simulink model "ADU_Integration_Y2016_simulation"  (R2016b)
settings: Solver=FixedStepDiscrete  StartTime=240  StopTime=300  FixedStep=0.01  RelTol=1e-3  EnableMultiTasking=on
PostLoadFcn:
  | , if any(exist('dsrtsu_mdlpostloadfcn', 'file') == [2, 3, 6]), try dsrtsu_mdlpostloadfcn('Execute', bdroot); catch fprintf('Error in PostLoadFcn (dsrtsu_mdlpostloadfcn) for model "%s":\n %s\n', bdroot, lasterr); end, end,
InitFcn:
  | load 'data/chi2_dat';
  | load 'data/innerLine_struct';
  | load 'data/middleLine_struct';
  | load 'data/outerLine_struct';
  | load 'data/innerLine';
  | load 'data/middleLine';
  | load 'data/outerLine';
  | load 'data/landmarks_patac_schimmel_ccw';
  | load 'data/patac_navi_array';
  | load 'data/sensor';
  | load 'data/map_struct';
  | addpath map_src
  | Integration_Parameter;
  | load 'TestData_001';
values from neighbouring files (symbols this model uses):
  TestData_001 =     [TestData_001.mat]
undefined symbols (not defined in the file or in its folder): a, chi2_dat, innerLine, landmarks_patac_schimmel_ccw, middleLine, outerLine, patac_navi_array, StartNum
libraries: simulink x36, rtican x1
(part 10 of 20)

== stateflow chart ADU_Integration_Y2016_simulation/Fusion_Model/Fusion_Block/Global_Fusion/Fusion_Center ==
  state Fusion_Main [parallel]
    settings: executionOrder=2
    state D
    (default) -> D
    D -> (junction 4544)
    (junction 4544) -> (junction 4092) : {
        | FusDataIni();
        | FusTrackPredict();
        | MeasurementsGen();
        | FusTrackUpdate();
        | FusTrackIni();
        | }
    (junction 4092) -> (junction 4091) : {
        | Num_Trg=TrackCounter;
        | LastCalTime=Sensor_sampleTime;
        | }
    (junction 4091) -> (junction 4983) [order 1] : [RollCount<=2]
    (junction 4091) -> (junction 4987) [order 2] : {
        | RollCount=0;
        | }
    (junction 4983) -> (junction 4985) : {
        | RollCount++;
        | }
    (junction 4985) -> (junction 4987)
    (junction 4987) -> Fusion_Main
  state Set_Data_Source(data) [function]
    (default) -> (junction 1370)
    (junction 1370) -> (junction 1371) : {
        | DataSource = data;
        | }
  state DataSet [parallel]
    settings: executionOrder=1
    state C
    (default) -> C
    C -> (junction 5010)
    (junction 5010) -> (junction 5011) [order 1] : cal%Camera_Update
    (junction 5010) -> (junction 5015) [order 2]
    (junction 5011) -> (junction 5013) : {
        | Set_Data_Source(1);
        | Set_sampleTime(Camera_RxTime);
        | }
    (junction 5015) -> (junction 5017) [order 1] : cal1%SRR Update
    (junction 5015) -> (junction 5021) [order 2]
    (junction 5017) -> (junction 5019) : {
        | Set_Data_Source(3);
        | Set_sampleTime(SRR_RxTime);
        | }
    (junction 5021) -> (junction 5023) [order 1] : cal2%ESR Update
    (junction 5021) -> (junction 5027) [order 2]
    (junction 5023) -> (junction 5025) : {
        | Set_Data_Source(2);
        | Set_sampleTime(ESR_RxTime);
        | }
    (junction 5025) -> (junction 5027)
    (junction 5019) -> (junction 5025)
    (junction 5013) -> (junction 5019)
    (junction 5027) -> (junction 5047)
    (junction 5047) -> DataSet
  state Set_sampleTime(data) [function]
    (default) -> (junction 1375)
    (junction 1375) -> (junction 1376) : {
        | Sensor_sampleTime = data;
        | }
  state FusDataIni [function]
    (default) -> (junction 4085)
    (junction 4085) -> (junction 4086) : {
        | deltaT=Sensor_sampleTime-LastCalTime;ExistID=0;
        | k=0;n=0;m=0;FusDataOut=0;
        | FusDataInternal=0;%Initial step
        | MeasureData=0;MD_Exist=0;UpdateTrackFlag=0;
        | DelectTrackFlag=0;TrackCounter=0;Num_Out=0;ScoreFlag=0;
        | }
    (junction 4086) -> (junction 4087)
  state FusTrackPredict [function]
    state [RangeX,VelX,RangeY,VelY,P11,P12,P13,P14,P21,P22,P23,P24,P31,P32,P33,P34,P41,P42,P43,... [function]
      P44] = Forecast(Pre_x,Pre_vx,Pre_y,Pre_vy,deltaT,pre_p11,pre_p12,pre_p13,pre_p14,pre_p21,...
      pre_p22,pre_p23,pre_p24,pre_p31,pre_p32,pre_p33,pre_p34,pre_p41,pre_p42,pre_p43,pre_p44)
    (default) -> (junction 3932)
    (junction 3932) -> (junction 3933) [order 1] : [k<Num_Trg]
    (junction 3933) -> (junction 3934) [order 1] : [FusDataInternal_temp[k][0]!=0]
    (junction 3935) -> (junction 3932) : {
        | k++;
        | }
    (junction 3932) -> (junction 3937) [order 2] : {
        | Num_Trg=n;
        | n=0;
        | }
    (junction 3933) -> (junction 3935) [order 2]
    (junction 3934) -> (junction 3936) : {
        | [FusDataInternal[n][1],FusDataInternal[n][2],FusDataInternal[n][3],FusDataInternal[n][4],FusDataInternal[n][11],FusDataInternal[n][12],FusDataInternal[n][13],FusDataInternal[n][14],...
        | FusDataInternal[n][15],FusDataInternal[n][16],FusDataInternal[n][17],FusDataInternal[k][18],FusDataInternal[k][19],FusDataInternal[k][20],FusDataInternal[n][21],FusDataInternal[n][22],...
        | FusDataInternal[n][23],FusDataInternal[n][24],FusDataInternal[n][25],FusDataInternal[n][26]]=Forecast(FusDataInternal_temp[k][1],FusDataInternal_temp[k][2],FusDataInternal_temp[k][3],...
        | FusDataInternal_temp[k][4],deltaT,FusDataInternal_temp[k][11],FusDataInternal_temp[k][12],FusDataInternal_temp[k][13],FusDataInternal_temp[k][14],FusDataInternal_temp[k][15],FusDataInternal_temp[k][16],...
        | FusDataInternal_temp[k][17],FusDataInternal_temp[k][18],FusDataInternal_temp[k][19],FusDataInternal_temp[k][20],FusDataInternal_temp[k][21],FusDataInternal_temp[k][22],FusDataInternal_temp[k][23],...
        | FusDataInternal_temp[k][24],FusDataInternal_temp[k][25],FusDataInternal_temp[k][26]);%All fusion targets forecast,after this step, target number in FusDataInternal is the same as last calculation, but forecast with delta time
        | FusDataInternal[n][0]=FusDataInternal_temp[k][0];FusDataInternal[n][5]=FusDataInternal_temp[k][5];FusDataInternal[n][6]=FusDataInternal_temp[k][6];FusDataInternal[n][7]=FusDataInternal_temp[k][7];...
        | FusDataInternal[n][8]=FusDataInternal_temp[k][8];FusDataInternal[n][9]=FusDataInternal_temp[k][9];FusDataInternal[n][10]=FusDataInternal_temp[k][10];
        | FusDataInternal[n][27]=FusDataInternal_temp[k][27];FusDataInternal[n][28]=FusDataInternal_temp[k][28];FusDataInternal[n][29]=FusDataInternal_temp[k][29];
        | FusDataInternal[n][30]=FusDataInternal_temp[k][30];FusDataInternal[n][31]=FusDataInternal_temp[k][31];
        | n++;
        | }
    (junction 3936) -> (junction 3935)
  state MeasurementsGen [function]
    (default) -> (junction 4061) : {
        | k=0;
        | FusDataInternal_temp=0;
        | }
    (junction 4062) -> (junction 4063) [order 1] : [(k<64) ]
    (junction 4061) -> (junction 4062) [order 1] : [DataSource==2]%ESR Data Update
    (junction 4067) -> (junction 4062) : {
        | k++;
        | }
    (junction 4062) -> (junction 4069) [order 2]
    (junction 4063) -> (junction 4067) : {
        | MeasureData[k][0]=ESRData[k][0];
        | MeasureData[k][1]=ESRData[k][1];
        | MeasureData[k][2]=ESRData[k][2];
        | MeasureData[k][3]=0;MeasureData[k][4]=0;
        | MeasureData[k][5]=0;MeasureData[k][6]=0.1;
        | MeasureData[k][7]=0;MeasureData[k][8]=0;
        | MeasureData[k][9]=0.6;
        | }
    (junction 4061) -> (junction 4064) [order 2]
    (junction 4064) -> (junction 4547) [order 1] : [DataSource==3]%SRR Data Update
    (junction 4547) -> (junction 4549) [order 1] : [(k<40)]
    (junction 4551) -> (junction 4547) : {
        | k++;
        | }
    (junction 4064) -> (junction 4560) [order 2]
    (junction 4547) -> (junction 4068) [order 2]
    (junction 4549) -> (junction 4551) : {
        | MeasureData[k][0]=SRRData[k][0];
        | MeasureData[k][1]=SRRData[k][1];
        | MeasureData[k][2]=SRRData[k][2];
        | MeasureData[k][3]=SRRData[k][3];
        | MeasureData[k][4]=0;MeasureData[k][5]=0;
        | MeasureData[k][6]=1;MeasureData[k][7]=0;
        | MeasureData[k][8]=0;MeasureData[k][9]=1;
        | }
    (junction 4560) -> (junction 4065) [order 1] : [(k<25)]
    (junction 4066) -> (junction 4560) : {
        | k++;
        | }
    (junction 4065) -> (junction 4066) : {
        | MeasureData[k][0]=CameraData[k][0];MeasureData[k][1]=CameraData[k][1];
        | MeasureData[k][2]=CameraData[k][2];MeasureData[k][3]=CameraData[k][7];
        | MeasureData[k][4]=CameraData[k][4];MeasureData[k][5]=CameraData[k][3];
        | MeasureData[k][6]=0.3*CameraData[k][1];MeasureData[k][7]=0;
        | MeasureData[k][8]=0;MeasureData[k][9]=0.01;
        | }
    (junction 4560) -> (junction 4565) [order 2]
    (junction 4068) -> (junction 4565)
    (junction 4069) -> (junction 4068)
    (junction 4565) -> (junction 4070)
  state FusTrackUpdate [function]
    state [RangeX,VelX,RangeY,VelY,P11,P12,P13,P14,P21,P22,P23,P24,P31,P32,P33,P34,P41,P42,P43,... [function]
      P44] = Update(Pre_x,Pre_vx,Pre_y,Pre_vy,Mea_x,Mea_y,pre_p11,pre_p12,pre_p13,pre_p14,pre_p21,...
      pre_p22,pre_p23,pre_p24,pre_p31,pre_p32,pre_p33,pre_p34,pre_p41,pre_p42,pre_p43,pre_p44,R11,R12,R21,R22)
    state step1 [function]
      state Association_Update_step1 [function]
        (default) -> (junction 4252)
        (junction 4252) -> (junction 4253) [order 1] : [DataSource!=1]%Not Camera
        (junction 4253) -> (junction 4573) [order 1] : [DataSource!=2]%SRR
        (junction 4252) -> (junction 4254) [order 2] : {
            | ExistID=FusDataInternal[k][29];
            | }
        (junction 4253) -> (junction 4255) [order 2] : {
            | ExistID=FusDataInternal[k][27];
            | }
        (junction 4573) -> (junction 4575) : {
            | ExistID=FusDataInternal[k][28];
            | }
        (junction 4255) -> (junction 4254)
        (junction 4575) -> (junction 4255)
        (junction 4254) -> (junction 4257)
        (junction 4257) -> (junction 4256) [order 1] : [n<64]
        (junction 4256) -> (junction 4258) [order 1] : [(MeasureData[n][0]==ExistID) &&(MeasureData[n][10] == 0) &&(MeasureData[n][0] != 0)]
        (junction 4259) -> (junction 4257) : {
            | n++;
            | }
        (junction 4256) -> (junction 4259) [order 2]
        (junction 4257) -> (junction 4260) [order 2]
          settings: description=%not found last updata message
        (junction 4258) -> (junction 4261) : {
            | MD_Exist=MDCal(MeasureData[n][1],MeasureData[n][2],...
            | FusDataInternal[k][1],FusDataInternal[k][3],FusDataInternal[k][11],...
            | FusDataInternal[k][12],FusDataInternal[k][13],FusDataInternal[k][14],FusDataInternal[k][15],...
            | FusDataInternal[k][16],FusDataInternal[k][17],FusDataInternal[k][18],FusDataInternal[k][19],...
            | FusDataInternal[k][20],FusDataInternal[k][21],FusDataInternal[k][22],FusDataInternal[k][23],...
            | FusDataInternal[k][24],FusDataInternal[k][25],FusDataInternal[k][26],MeasureData[n][6],...
            | MeasureData[n][7],MeasureData[n][8],MeasureData[n][9]);
            | }
        (junction 4261) -> (junction 4260) [order 2] : %Not find exist measurement last time
          settings: description=%last measurement is out of range
        (junction 4261) -> (junction 4262) [order 1] : [MD_Exist<MD_Calib]
        (junction 4260) -> (junction 4263)
        (junction 4262) -> (junction 4727) : {
            | MeasureFoundNum=n;
            | [FusDataInternal_temp[k][1],FusDataInternal_temp[k][2],FusDataInternal_temp[k][3],FusDataInternal_temp[k][4],...
            | FusDataInternal_temp[k][11],FusDataInternal_temp[k][12],FusDataInternal_temp[k][13],FusDataInternal_temp[k][14],...
            | FusDataInternal_temp[k][15],FusDataInternal_temp[k][16],FusDataInternal_temp[k][17],FusDataInternal_temp[k][18],...
            | FusDataInternal_temp[k][19],FusDataInternal_temp[k][20],FusDataInternal_temp[k][21],FusDataInternal_temp[k][22],...
            | FusDataInternal_temp[k][23],FusDataInternal_temp[k][24],FusDataInternal_temp[k][25],FusDataInternal_temp[k][26]]=...
            | Update(FusDataInternal[k][1],FusDataInternal[k][2],FusDataInternal[k][3],FusDataInternal[k][4],...
            | MeasureData[MeasureFoundNum][1],MeasureData[MeasureFoundNum][2],...
            | FusDataInternal[k][11],FusDataInternal[k][12],FusDataInternal[k][13],FusDataInternal[k][14],...
            | FusDataInternal[k][15],FusDataInternal[k][16],FusDataInternal[k][17],FusDataInternal[k][18],...
            | FusDataInternal[k][19],FusDataInternal[k][20],FusDataInternal[k][21],FusDataInternal[k][22],...
            | FusDataInternal[k][23],FusDataInternal[k][24],FusDataInternal[k][25],FusDataInternal[k][26],...
            | MeasureData[MeasureFoundNum][6],MeasureData[MeasureFoundNum][7],MeasureData[MeasureFoundNum][8],MeasureData[MeasureFoundNum][9]);
            | FusDataInternal_temp[k][0]=FusDataInternal[k][0];FusDataInternal_temp[k][5]=FusDataInternal[k][5];FusDataInternal_temp[k][6]=FusDataInternal[k][6];
            | FusDataInternal_temp[k][8]=FusDataInternal[k][8];FusDataInternal_temp[k][9]=FusDataInternal[k][9];
            | FusDataInternal_temp[k][10]=FusDataInternal[k][10];FusDataInternal_temp[k][27]=FusDataInternal[k][27];
            | FusDataInternal_temp[k][28]=FusDataInternal[k][28];FusDataInternal_temp[k][29]=FusDataInternal[k][29];
            | FusDataInternal_temp[k][30]=FusDataInternal[k][30];FusDataInternal_temp[k][31]=FusDataInternal[k][31];
            | %Update track k with measurement (MeasureFoundNum)
            | UpdateTrackFlag[k]=1;%Track k is marked as updated
            | MeasureData[MeasureFoundNum][10]=1;%Measurement is marked as used
            | }
        (junction 4727) -> (junction 4728) [order 1] : [DataSource==1]%Camera
        (junction 4727) -> (junction 4264) [order 2] : {
            | FusDataInternal_temp[k][7]=FusDataInternal[k][7];
            | FusDataInternal_temp[k][6]=FusDataInternal[k][6];
            | }
        (junction 4728) -> (junction 4731) : {
            | FusDataInternal_temp[k][7]=MeasureData[MeasureFoundNum][10];
            | FusDataInternal_temp[k][6]=MeasureData[MeasureFoundNum][4];
            | }
        (junction 4264) -> (junction 4263)
        (junction 4731) -> (junction 4264)
        (junction 4263) -> (junction 4265)
      (default) -> (junction 4235) : {
          | k=0;ExistID=0;
          | %Gating and Association Step
          | }
      (junction 4235) -> (junction 4236) [order 1] : [k<Num_Trg]
      (junction 4240) -> (junction 4235) : {
          | n=0;k++;
          | MeasureFoundNum=0;
          | }
      (junction 4235) -> (junction 4239) [order 2]
      (junction 4236) -> (junction 4237) : {Association_Update_step1();}
      (junction 4237) -> (junction 4238) [order 1] : [UpdateTrackFlag[k]==1]
      (junction 4237) -> (junction 4240) [order 2]
      (junction 4238) -> (junction 4241) : {
          | UpdateSourceID();
          | }
      (junction 4241) -> (junction 4240)
    state step2 [function]
      state Association_Update_step2 [function]
        state gating [function]
          (default) -> (junction 4342)
          (junction 4342) -> (junction 4343) [order 1] : [m<64]
          (junction 4343) -> (junction 4344) [order 1] : [(MeasureData[m][0] !=0) &&...
              |  (MeasureData[m][10]==0)]
          (junction 4354) -> (junction 4342) : {
              | m++;
              | }
          (junction 4342) -> (junction 4351) [order 2]
          (junction 4343) -> (junction 4354) [order 2]
          (junction 4344) -> (junction 4348)
          (junction 4348) -> (junction 4346) [order 1] : [(MeasureData[m][1] <= FusDataInternal[k][1] + Rx3xgm) && ...
              |  (MeasureData[m][1] >= FusDataInternal[k][1] - Rx3xgm)  &&...
              |  (MeasureData[m][2] <= FusDataInternal[k][3] + Ry3xgm) && ...
              |  (MeasureData[m][2] >= FusDataInternal[k][3] - Ry3xgm)]
          (junction 4348) -> (junction 4355) [order 2]
          (junction 4346) -> (junction 4349) : {
              | MD_k_m=MDCal(MeasureData[m][1],MeasureData[m][2],...
              | FusDataInternal[k][1],FusDataInternal[k][3],FusDataInternal[k][11],...
              | FusDataInternal[k][12],FusDataInternal[k][13],FusDataInternal[k][14],FusDataInternal[k][15],...
              | FusDataInternal[k][16],FusDataInternal[k][17],FusDataInternal[k][18],FusDataInternal[k][19],...
              | FusDataInternal[k][20],FusDataInternal[k][21],FusDataInternal[k][22],FusDataInternal[k][23],...
              | FusDataInternal[k][24],FusDataInternal[k][25],FusDataInternal[k][26],MeasureData[m][6],...
              | MeasureData[m][7],MeasureData[m][8],MeasureData[m][9]);
              | }
          (junction 4349) -> (junction 4350) [order 1] : [MD_k_m<MD_min]
          (junction 4349) -> (junction 4352) [order 2]
          (junction 4350) -> (junction 4353) : {
              | MD_min=MD_k_m;
              | MeasureFoundFlag=1;
              | MeasureFoundNum=m;
              | }
          (junction 4353) -> (junction 4352)
          (junction 4352) -> (junction 4355)
          (junction 4355) -> (junction 4354)
        (default) -> (junction 4300)
        (junction 4300) -> (junction 4301) [order 1] : [(DataSource==2) || (DataSource==3)]%Radar(ESR and SRR)
        (junction 4300) -> (junction 4302) [order 2] : {
            | Ry3xgm=1;
            | }
        (junction 4301) -> (junction 4589) : {
            | Ry3xgm=1;
            | }
        (junction 4302) -> (junction 4303) [order 1] : [FusDataInternal[k][1] >= 0]
        (junction 4589) -> (junction 4590) [order 1] : [FusDataInternal[k][1]>=0]
        (junction 4302) -> (junction 4304) [order 2] : {
            | Rx3xgm=-0.3*FusDataInternal[k][1]+1;
            | }
        (junction 4589) -> (junction 4306) [order 2] : {
            | Rx3xgm=-0.15*FusDataInternal[k][1]+1;
            | }
        (junction 4303) -> (junction 4305) : {
            | Rx3xgm=0.3*FusDataInternal[k][1]+1;
            | }
        (junction 4590) -> (junction 4592) : {
            | Rx3xgm=0.15*FusDataInternal[k][1]+1;
            | }
        (junction 4305) -> (junction 4304)
        (junction 4306) -> (junction 4305)
        (junction 4592) -> (junction 4306)
        (junction 4304) -> (junction 4307)
        (junction 4307) -> (junction 4308) [order 1] : [UpdateTrackFlag[k]==0]
        (junction 4307) -> (junction 4315) [order 2]
        (junction 4308) -> (junction 4309) : {
            | gating();
            | }
        (junction 4309) -> (junction 4310) [order 1] : [MeasureFoundFlag ==1]
        (junction 4309) -> (junction 4311) [order 2] : {
            | UpdateTrackFlag[k]=0;
            | %Track k is not found updata measurement
            | }
        (junction 4310) -> (junction 4740) : {
            | [FusDataInternal_temp[k][1],FusDataInternal_temp[k][2],FusDataInternal_temp[k][3],FusDataInternal_temp[k][4],...
            | FusDataInternal_temp[k][11],FusDataInternal_temp[k][12],FusDataInternal_temp[k][13],FusDataInternal_temp[k][14],...
            | FusDataInternal_temp[k][15],FusDataInternal_temp[k][16],FusDataInternal_temp[k][17],FusDataInternal_temp[k][18],...
            | FusDataInternal_temp[k][19],FusDataInternal_temp[k][20],FusDataInternal_temp[k][21],FusDataInternal_temp[k][22],...
            | FusDataInternal_temp[k][23],FusDataInternal_temp[k][24],FusDataInternal_temp[k][25],FusDataInternal_temp[k][26]]=...
            | Update(FusDataInternal[k][1],FusDataInternal[k][2],FusDataInternal[k][3],FusDataInternal[k][4],...
            | MeasureData[MeasureFoundNum][1],MeasureData[MeasureFoundNum][2],...
            | FusDataInternal[k][11],FusDataInternal[k][12],FusDataInternal[k][13],FusDataInternal[k][14],...
            | FusDataInternal[k][15],FusDataInternal[k][16],FusDataInternal[k][17],FusDataInternal[k][18],...
            | FusDataInternal[k][19],FusDataInternal[k][20],FusDataInternal[k][21],FusDataInternal[k][22],...
            | FusDataInternal[k][23],FusDataInternal[k][24],FusDataInternal[k][25],FusDataInternal[k][26],...
            | MeasureData[MeasureFoundNum][6],MeasureData[MeasureFoundNum][7],MeasureData[MeasureFoundNum][8],MeasureData[MeasureFoundNum][9]);
            | FusDataInternal_temp[k][0]=FusDataInternal[k][0];FusDataInternal_temp[k][5]=FusDataInternal[k][5];FusDataInternal_temp[k][6]=FusDataInternal[k][6];
            | FusDataInternal_temp[k][8]=FusDataInternal[k][8];FusDataInternal_temp[k][9]=FusDataInternal[k][9];
            | FusDataInternal_temp[k][10]=FusDataInternal[k][10];FusDataInternal_temp[k][27]=FusDataInternal[k][27];
            | FusDataInternal_temp[k][28]=FusDataInternal[k][28];FusDataInternal_temp[k][29]=FusDataInternal[k][29];
            | FusDataInternal_temp[k][30]=FusDataInternal[k][30];FusDataInternal_temp[k][31]=FusDataInternal[k][31];%Update track k with measurement (MeasureFoundNum)
            | UpdateTrackFlag[k]=1;%Track k is marked as updated
            | MeasureData[MeasureFoundNum][10]=1;%Measurement is marked as used
            | }
        (junction 4311) -> (junction 4312) [order 1] : [c<32]
        (junction 4313) -> (junction 4311) : {c++;}
        (junction 4311) -> (junction 4316) [order 2] : {
            | c=0;
            | }
        (junction 4312) -> (junction 4313) : {
            | FusDataInternal_temp[k][c]=...
            | FusDataInternal[k][c];
            | }
        (junction 4740) -> (junction 4738) [order 1] : [DataSource==1]%Camera
        (junction 4738) -> (junction 4737) : {
            | FusDataInternal_temp[k][7]=MeasureData[MeasureFoundNum][10];
            | FusDataInternal_temp[k][6]=MeasureData[MeasureFoundNum][4];
            | }
        (junction 4740) -> (junction 4314) [order 2] : {
            | FusDataInternal_temp[k][7]=FusDataInternal[k][7];
            | FusDataInternal_temp[k][6]=FusDataInternal[k][6];
            | }
        (junction 4737) -> (junction 4314)
        (junction 4314) -> (junction 4316)
        (junction 4316) -> (junction 4315)
        (junction 4315) -> (junction 4317)
      (default) -> (junction 4285) : {
          | k=0;MD_min=8000;m=0;TrackCounter=0;
          | Rx3xgm=0;Ry3xgm=0;%Gating and Association Step
          | }
      (junction 4285) -> (junction 4286) [order 1] : [k<Num_Trg]
      (junction 4286) -> (junction 4287) [order 1] : [UpdateTrackFlag[k]==0]
      (junction 4288) -> (junction 4285) : {
          | k++;MeasureFoundFlag=0;m=0;
          | MD_min=8000;
          | }
      (junction 4285) -> (junction 4290) [order 2]
      (junction 4286) -> (junction 4288) [order 2]
      (junction 4287) -> (junction 4289) : {
          | Association_Update_step2();
          | UpdateSourceID();
          | }
      (junction 4289) -> (junction 4288)
    state MD = MDCal(MeasureRx,MeasureRy,PredictRx,PredictRy,P11,P12,... [function]
      P13,P14,P21,P22,P23,P24,P31,P32,P33,P34,P41,P42,P43,P44,R11,R12,R21,R22)
    state step3 [function]
      state FusTrackManagement [function]
        state ExistScoreCal [function]
          state OutSRRFOV= OutSRRFOV [function]
            (default) -> (junction 4680)
            (junction 4680) -> (junction 4710) [order 1] : [(FusDataInternal_temp[k][1]>=0)]
            (junction 4710) -> (junction 4712) [order 1] : [((FusDataInternal_temp[k][1])*(FusDataInternal_temp[k][1])+(FusDataInternal_temp[k][3])*(FusDataInternal_temp[k][3])>=60*60) && ...
                | ((FusDataInternal_temp[k][3]<FusDataInternal_temp[k][1]*tan(20*3.14/180)) && (FusDataInternal_temp[k][3]>-1*FusDataInternal_temp[k][1]*tan(20*3.14/180)))]
            (junction 4680) -> (junction 4709) [order 2]
            (junction 4710) -> (junction 4716) [order 2]
            (junction 4712) -> (junction 4714) : {
                | OutSRRFOV=1;
                | }
            (junction 4716) -> (junction 4709)
            (junction 4709) -> (junction 4719) : {
                | OutSRRFOV=0;
                | }
            (junction 4714) -> (junction 4719)
            (junction 4719) -> (junction 4722)
          state OutESRFOV= OutESRFOV [function]
            (default) -> (junction 4636)
            (junction 4636) -> (junction 4637) [order 1] : [(FusDataInternal_temp[k][1]<=0)]%Source is ESR and out of FOV
            (junction 4636) -> (junction 4638) [order 2]
            (junction 4637) -> (junction 4639)
            (junction 4638) -> (junction 4655) [order 1] : [(FusDataInternal_temp[k][1]>=60)]%LRR Mode
            (junction 4655) -> (junction 4639) [order 1] : [(FusDataInternal_temp[k][3]>FusDataInternal_temp[k][1]*tan(10*3.14/180)) || ...
                | (FusDataInternal_temp[k][3]<-1*FusDataInternal_temp[k][1]*tan(10*3.14/180))]
            (junction 4638) -> (junction 4657) [order 2]
            (junction 4655) -> (junction 4661) [order 2] : {
                | OutESRFOV = 0;
                | }
            (junction 4639) -> (junction 4641) : {
                | OutESRFOV = 1;
                | }
            (junction 4657) -> (junction 4669) [order 1] : [(FusDataInternal_temp[k][3]>FusDataInternal_temp[k][1]*tan(45*3.14/180)) || ...
                | (FusDataInternal_temp[k][3]<-1*FusDataInternal_temp[k][1]*tan(45*3.14/180))]%MRR Mode
            (junction 4657) -> (junction 4640) [order 2] : {
                | OutESRFOV = 0;
                | }
            (junction 4669) -> (junction 4670) : {
                | OutESRFOV = 1;
                | }
            (junction 4670) -> (junction 4640)
            (junction 4661) -> (junction 4670)
            (junction 4641) -> (junction 4661)
            (junction 4640) -> (junction 4642)
          state OutCameraFOV= OutCameraFOV [function]
            (default) -> (junction 4608)
            (junction 4608) -> (junction 4622) [order 1] : [(FusDataInternal_temp[k][1]<=0)]%Source is Camera and out of FOV
            (junction 4608) -> (junction 4628) [order 2]
            (junction 4622) -> (junction 4630)
            (junction 4628) -> (junction 4630) [order 1] : [(FusDataInternal_temp[k][3]>FusDataInternal_temp[k][1]*tan(20*3.14/180)) || ...
                | (FusDataInternal_temp[k][3]<-1*FusDataInternal_temp[k][1]*tan(20*3.14/180))]
            (junction 4628) -> (junction 4610) [order 2] : {
                | OutCameraFOV = 0;
                | }
            (junction 4630) -> (junction 4624) : {
                | OutCameraFOV = 1;
                | }
            (junction 4624) -> (junction 4610)
            (junction 4610) -> (junction 4612)
          state Blocked = CameraBlocked [function]
            (default) -> (junction 4437) : {
                | h = 0;
                | }
            (junction 4435) -> (junction 5000) [order 1] : [(MeasureData[h][0]!=0)&&...
                | (MeasureData[h][1]>0)]
            (junction 5000) -> (junction 4436) [order 1] : [(FusDataInternal_temp[k][1] >MeasureData[h][1]+2)&&...
                | (FusDataInternal_temp[k][1] <MeasureData[h][1]+20)&&...
                | (FusDataInternal_temp[k][3] <MeasureData[h][2] +1)&&...
                | (FusDataInternal_temp[k][3] >MeasureData[h][2] -1)]
            (junction 4437) -> (junction 4435) [order 1] : [h<25]
            (junction 4435) -> (junction 4438) [order 2]
            (junction 5000) -> (junction 5002) [order 2]
            (junction 4436) -> (junction 4440) : {
                | Blocked = 1;
                | }
            (junction 4438) -> (junction 4437) : {
                | h++;
                | }
            (junction 4437) -> (junction 4439) [order 2] : {
                | Blocked = 0;
                | }
            (junction 5002) -> (junction 4438)
            (junction 4440) -> (junction 4439)
            (junction 4439) -> (junction 4441)
          state ScoreIncrease [function]
            state CameraIncrease [function]
              (default) -> (junction 4883)
              (junction 4883) -> (junction 4886) : {
                  | FusDataInternal_temp[k][30]=...
                  | FusDataInternal_temp[k][30]+CameraScoreIn;
                  | FusDataInternal_temp[k][32]=7;
                  | }
              (junction 4886) -> (junction 4889)
            state SRRIncrease [function]
              (default) -> (junction 4901)
              (junction 4901) -> (junction 4902) : {
                  | FusDataInternal_temp[k][30]=...
                  | FusDataInternal_temp[k][30]+SRRScoreIn;
                  | FusDataInternal_temp[k][32]=8;
                  | }
              (junction 4902) -> (junction 4903)
            state ESRIncrease [function]
              (default) -> (junction 4908)
              (junction 4908) -> (junction 4914) [order 1] : [(FusDataInternal_temp[k][3]<10) &&...
                  |  (FusDataInternal_temp[k][3]>-10)]
              (junction 4914) -> (junction 4920) [order 1] : [(FusDataInternal_temp[k][3]<5) &&...
                  |  (FusDataInternal_temp[k][3]>-5)]
              (junction 4908) -> (junction 4909) [order 2] : {
                  | FusDataInternal_temp[k][30]=...
                  | FusDataInternal_temp[k][30]+ESRScoreIn;
                  | FusDataInternal_temp[k][32]=91;
                  | %Lateral Range is Far
                  | }
              (junction 4914) -> (junction 4924) [order 2] : {
                  | FusDataInternal_temp[k][30]=...
                  | FusDataInternal_temp[k][30]+ESRScoreIn;
                  | FusDataInternal_temp[k][32]=92;
                  | %Lateral Range is Middle
                  | }
              (junction 4920) -> (junction 4922) : {
                  | FusDataInternal_temp[k][30]=...
                  | FusDataInternal_temp[k][30]+ESRScoreIn;
                  | FusDataInternal_temp[k][32]=93;
                  | %Lateral Range is Near
                  | }
              (junction 4924) -> (junction 4909)
              (junction 4922) -> (junction 4924)
              (junction 4909) -> (junction 4910)
            (default) -> (junction 4755)
            (junction 4755) -> (junction 4762) [order 1] : [DataSource!=1]
            (junction 4762) -> (junction 4768) [order 1] : [DataSource!=2]
            (junction 4755) -> (junction 4764) [order 2] : {
                | CameraIncrease();
                | %Camera
                | }
            (junction 4762) -> (junction 4766) [order 2] : {
                | ESRIncrease();
                | %ESR
                | }
            (junction 4768) -> (junction 4771) : {
                | SRRIncrease();
                | %SRR
                | }
            (junction 4766) -> (junction 4764)
            (junction 4771) -> (junction 4766)
            (junction 4764) -> (junction 4775)
          state ScoreDecrease [function]
            (default) -> (junction 4778)
            (junction 4779) -> (junction 4780) [order 1] : [DataSource!=2]
            (junction 4778) -> (junction 4779) [order 1] : [DataSource!=1]
            (junction 4779) -> (junction 4782) [order 2] : {
                | FusDataInternal_temp[k][30]=...
                | FusDataInternal_temp[k][30]-ESRScoreDe;
                | FusDataInternal_temp[k][32]=13;
                | %ESR
                | }
            (junction 4780) -> (junction 4783) : {
                | FusDataInternal_temp[k][30]=...
                | FusDataInternal_temp[k][30]-SRRScoreDe;
                | FusDataInternal_temp[k][32]=14;
                | %SRR
                | }
            (junction 4778) -> (junction 4973) [order 2]
            (junction 4973) -> (junction 4975) [order 1] : [((FusDataInternal_temp[k][3]<3) && (FusDataInternal_temp[k][3]>-3))&&...
                | FusDataInternal_temp[k][1]<30]
            (junction 4973) -> (junction 4781) [order 2] : {
                | FusDataInternal_temp[k][30]=...
                | FusDataInternal_temp[k][30]-CameraFarScoreDe;
                | FusDataInternal_temp[k][32]=11;
                | %Camera
                | }
            (junction 4975) -> (junction 4977) : {
                | FusDataInternal_temp[k][30]=...
                | FusDataInternal_temp[k][30]-CameraNearScoreDe;
                | FusDataInternal_temp[k][32]=12;
                | %Camera
                | }
            (junction 4783) -> (junction 4782)
            (junction 4782) -> (junction 4977)
            (junction 4977) -> (junction 4781)
            (junction 4781) -> (junction 4784)
          (default) -> (junction 4401)
          (junction 4401) -> (junction 4400) [order 1] : [UpdateTrackFlag[k]==1]
          (junction 4400) -> (junction 4404) : {
              | ScoreIncrease();
              | ScoreFlag=6;
              | }
          (junction 4401) -> (junction 4402) [order 2]
          (junction 4402) -> (junction 4403) [order 1] : [(DataSource==1) && (OutCameraFOV()==1)]%Source is Camera and out of FOV
          (junction 4402) -> (junction 4406) [order 2]
          (junction 4403) -> (junction 4410) : {
              | FusDataInternal_temp[k][32]=5;
              | }
          (junction 4406) -> (junction 4407) [order 1] : [(DataSource==1) && (FusDataInternal_temp[k][1]>0) &&(CameraBlocked() ==1)]% Source is Camera, but is blocked by other object
          (junction 4406) -> (junction 4599) [order 2]
          (junction 4407) -> (junction 4409) : {
              | FusDataInternal_temp[k][32]=4;
              | }
          (junction 4599) -> (junction 4601) [order 1] : [(DataSource==2) && (OutESRFOV()==1)]%Source is ESR and out of FOV
          (junction 4599) -> (junction 4673) [order 2]
          (junction 4601) -> (junction 4652) : {
              | FusDataInternal_temp[k][32]=3;
              | }
          (junction 4673) -> (junction 4675) [order 1] : [(DataSource==3) && (OutSRRFOV()==1)] % Source is SRR and out of FOV
          (junction 4673) -> (junction 4408) [order 2] : {
              | ScoreDecrease();
              | }
          (junction 4675) -> (junction 4724) : {
              | FusDataInternal_temp[k][32]=2;
              | }
          (junction 4404) -> (junction 4405) [order 1] : [FusDataInternal_temp[k][30]>18]
          (junction 4404) -> (junction 4411) [order 2]
          (junction 4405) -> (junction 4412) : {
              | FusDataInternal_temp[k][30]=18;
              | }
          (junction 4724) -> (junction 4408)
          (junction 4652) -> (junction 4724)
          (junction 4412) -> (junction 4411)
          (junction 4409) -> (junction 4652)
          (junction 4411) -> (junction 4410)
          (junction 4410) -> (junction 4409)
          (junction 4408) -> (junction 4413)
        state OutputTrack [function]
          (default) -> (junction 4452)
          (junction 4452) -> (junction 4453) [order 1] : [FusDataInternal_temp[k][31]==0]%Not a confirmed track
          (junction 4453) -> (junction 4454) [order 1] : [FusDataInternal_temp[k][30]<15]
          (junction 4452) -> (junction 4455) [order 2]
          (junction 4453) -> (junction 4456) [order 2] : {
              | FusDataInternal_temp[k][31]=1;
              | %New confirmed track
              | }
          (junction 4454) -> (junction 4464) : {
              | TrackCounter++;
              | }
          (junction 4456) -> (junction 4455)
          (junction 4455) -> (junction 4457) : {
              | FusDataOut[Num_Out][0]=FusDataInternal_temp[k][0];FusDataOut[Num_Out][1]=FusDataInternal_temp[k][1];
              | FusDataOut[Num_Out][2]=FusDataInternal_temp[k][2];FusDataOut[Num_Out][3]=FusDataInternal_temp[k][3];
              | FusDataOut[Num_Out][4]=FusDataInternal_temp[k][4];FusDataOut[Num_Out][5]=0;FusDataOut[Num_Out][6]=FusDataInternal_temp[k][6];FusDataOut[Num_Out][8]=0;
              | FusDataOut[Num_Out][7]=FusDataInternal_temp[k][7];%Type
              | FusDataOut[Num_Out][10]=FusDataInternal_temp[k][11];FusDataOut[Num_Out][11]=FusDataInternal_temp[k][12];
              | FusDataOut[Num_Out][12]=FusDataInternal_temp[k][13];FusDataOut[Num_Out][13]=FusDataInternal_temp[k][14];FusDataOut[Num_Out][14]=FusDataInternal_temp[k][15];
              | FusDataOut[Num_Out][15]=FusDataInternal_temp[k][16];FusDataOut[Num_Out][16]=FusDataInternal_temp[k][17];FusDataOut[Num_Out][17]=FusDataInternal_temp[k][18];
              | FusDataOut[Num_Out][18]=FusDataInternal_temp[k][19];FusDataOut[Num_Out][19]=FusDataInternal_temp[k][20];FusDataOut[Num_Out][20]=FusDataInternal_temp[k][21];
              | FusDataOut[Num_Out][21]=FusDataInternal_temp[k][22];FusDataOut[Num_Out][22]=FusDataInternal_temp[k][23];FusDataOut[Num_Out][23]=FusDataInternal_temp[k][24];
              | FusDataOut[Num_Out][24]=FusDataInternal_temp[k][25];FusDataOut[Num_Out][25]=FusDataInternal_temp[k][26];
              | %Select outputs signals from Internal to output
              | TrackCounter++;Num_Out++;
              | }
          (junction 4457) -> (junction 4458) [order 1] : [FusDataInternal_temp[k][30]<=15]
          (junction 4458) -> (junction 4459) [order 1] : [FusDataInternal_temp[k][30]<=9]
          (junction 4457) -> (junction 4460) [order 2] : {
              | FusDataOut[Num_Out-1][9]=3;
              | %High confidence
              | }
          (junction 4458) -> (junction 4461) [order 2] : {
              | FusDataOut[Num_Out-1][9]=2;
              | %Speculative
              | }
          (junction 4459) -> (junction 4462) : {
              | FusDataOut[Num_Out-1][9]=1;
              | %High Speculative
              | }
          (junction 4461) -> (junction 4460)
          (junction 4462) -> (junction 4461)
          (junction 4460) -> (junction 4463)
          (junction 4464) -> (junction 4463)
          (junction 4463) -> (junction 4465)
        state Del_InternalTrack [function]
          (default) -> (junction 4485) : {
              | DelectTrackFlag[k]=1;%mean that track need to delect
              | IDUsedFlag[FusDataInternal_temp[k][0]]=0;%Reflash ID Used Flag
              | }
          (junction 4485) -> (junction 4486) [order 1] : [c<32]
          (junction 4487) -> (junction 4485) : {c++;}
          (junction 4485) -> (junction 4488) [order 2] : {
              | c=0;
              | TrackCounter++;
              | }
          (junction 4486) -> (junction 4487) : {
              | FusDataInternal_temp[k][c]=0;
              | }
        (default) -> (junction 4386)
        (junction 4386) -> (junction 4387) : {
            | ExistScoreCal();
            | }
        (junction 4387) -> (junction 4388) [order 1] : [FusDataInternal_temp[k][30]>=0]%Marks >=0
        (junction 4387) -> (junction 4389) [order 2] : {
            | Del_InternalTrack();
            | }
        (junction 4388) -> (junction 4390) : {
            | OutputTrack();
            | }
        (junction 4390) -> (junction 4389)
        (junction 4389) -> (junction 4391)
      (default) -> (junction 4376) : {
          | k=0;TrackCounter=0;
          | }
      (junction 4376) -> (junction 4377) [order 1] : [k<Num_Trg]
      (junction 4379) -> (junction 4376) : {
          | k++;
          | }
      (junction 4376) -> (junction 4378) [order 2]
      (junction 4377) -> (junction 4379) : {
          | FusTrackManagement();
          | }
    state UpdateSourceID [function]
      (default) -> (junction 4521)
      (junction 4521) -> (junction 4522) [order 1] : [UpdateTrackFlag[k]==0]
      (junction 4522) -> (junction 4523) [order 1] : [DataSource !=1]
      (junction 4523) -> (junction 4578) [order 1] : [DataSource !=2]
      (junction 4521) -> (junction 4525) [order 2]
      (junction 4522) -> (junction 4529) [order 2] : {
          | FusDataInternal_temp[k][29] = -1;
          | }
      (junction 4523) -> (junction 4526) [order 2] : {
          | FusDataInternal_temp[k][27] = -1;
          | }
      (junction 4578) -> (junction 4580) : {
          | FusDataInternal_temp[k][28] = -1;
          | }
      (junction 4525) -> (junction 4524) [order 1] : [DataSource!=1]%ESR or SRR
      (junction 4524) -> (junction 4583) [order 1] : [DataSource!=2]%SRR
      (junction 4525) -> (junction 4527) [order 2] : {
          | FusDataInternal_temp[k][29]=MeasureData[MeasureFoundNum][0];
          | FusDataInternal_temp[k][9]=1;
          | }
      (junction 4524) -> (junction 4528) [order 2] : {
          | FusDataInternal_temp[k][27]=MeasureData[MeasureFoundNum][0];
          | FusDataInternal_temp[k][9]=2;
          | }
      (junction 4583) -> (junction 4585) : {
          | FusDataInternal_temp[k][28]=MeasureData[MeasureFoundNum][0];
          | FusDataInternal_temp[k][9]=3;
          | }
      (junction 4580) -> (junction 4526)
      (junction 4528) -> (junction 4527)
      (junction 4526) -> (junction 4529)
      (junction 4585) -> (junction 4528)
      (junction 4529) -> (junction 4585)
      (junction 4527) -> (junction 4530)
    (default) -> (junction 4095)
    (junction 4095) -> (junction 4096) : {
        | step1();
        | step2();
        | step3();
        | }
    (junction 4096) -> (junction 4097)
  state FusTrackIni [function]
    state InPathFlag =ESRInPathJudge(x,y,R) [function]
    (default) -> (junction 3890) : {
        | k=0;
        | n=0;
        | m=0;
        | }
    (junction 3890) -> (junction 3891) [order 1] : [k<64]
    (junction 3891) -> (junction 4929) [order 1] : [(MeasureData[k][0] !=0) && (MeasureData[k][10]==0)]
        | %Measurement k not association with fuse track
    (junction 4929) -> (junction 4958) [order 1] : [(DataSource==1) || (DataSource==3)]
    (junction 4958) -> (junction 3892)
    (junction 3892) -> (junction 3893) : {LastFusID++;}
    (junction 3893) -> (junction 3894) [order 1] : [LastFusID<127]
    (junction 3903) -> (junction 3890) : {
        | k++;
        | LoopError=0;
        | }
    (junction 3890) -> (junction 3902) [order 2]
    (junction 3891) -> (junction 3903) [order 2]
    (junction 4929) -> (junction 4933) [order 2] : {
        | InPathFlag=ESRInPathJudge(MeasureData[k][1],...
        | MeasureData[k][2],Path_Radius)
        | }%ESR Data
    (junction 4935) -> (junction 4958)
    (junction 3897) -> (junction 3892) : {
        | LoopError++;
        | }
    (junction 3893) -> (junction 3895) [order 2] : {LastFusID=1;}
    (junction 3894) -> (junction 3896)
    (junction 3895) -> (junction 3896)
    (junction 3896) -> (junction 3898)
    (junction 4933) -> (junction 4935) [order 1] : [(InPathFlag==1) && (DataSource==2)]
    (junction 3898) -> (junction 3897) [order 2] : [LoopError<126 && (IDUsedFlag[LastFusID]==1)]
    (junction 3898) -> (junction 3899) [order 1] : [IDUsedFlag[LastFusID]==0]
    (junction 4933) -> (junction 4961) [order 2]
    (junction 3898) -> (junction 3904) [order 3]
    (junction 3899) -> (junction 3900) : {
        | FusDataInternal_temp[TrackCounter][0]=LastFusID;IDUsedFlag[LastFusID]=1;
        | FusDataInternal_temp[TrackCounter][1]=MeasureData[k][1];FusDataInternal_temp[TrackCounter][2]=0;FusDataInternal_temp[TrackCounter][3]=MeasureData[k][2];
        | FusDataInternal_temp[TrackCounter][4]=0;
        | FusDataInternal_temp[TrackCounter][5]=0;FusDataInternal_temp[TrackCounter][6]=0;FusDataInternal_temp[TrackCounter][7]=0;
        | FusDataInternal_temp[TrackCounter][8]=0;FusDataInternal_temp[TrackCounter][9]=DataSource;
        | FusDataInternal_temp[TrackCounter][10]=1;
        | FusDataInternal_temp[TrackCounter][11]=1;FusDataInternal_temp[TrackCounter][16]=1;FusDataInternal_temp[TrackCounter][21]=1;FusDataInternal_temp[TrackCounter][26]=1;
        | FusDataInternal_temp[TrackCounter][30]=5;FusDataInternal_temp[TrackCounter][31]=0;
        | }
    (junction 3900) -> (junction 3901) [order 1] : [DataSource!=1]
    (junction 3901) -> (junction 4741) [order 1] : [DataSource!=2]
    (junction 3900) -> (junction 3905) [order 2] : {
        | FusDataInternal_temp[TrackCounter][29]=MeasureData[k][0];
        | FusDataInternal_temp[TrackCounter][6]=MeasureData[k][4];
        | FusDataInternal_temp[TrackCounter][7]=MeasureData[k][5];
        | TrackCounter++;
        | }
    (junction 3901) -> (junction 3906) [order 2] : {
        | FusDataInternal_temp[TrackCounter][27]=MeasureData[k][0];
        | TrackCounter++;
        | }
    (junction 4741) -> (junction 4743) : {
        | FusDataInternal_temp[TrackCounter][28]=MeasureData[k][0];
        | TrackCounter++;
        | }
    (junction 4961) -> (junction 3903)
    (junction 3904) -> (junction 4961)
    (junction 3905) -> (junction 3904)
    (junction 3906) -> (junction 3905)
    (junction 4743) -> (junction 3906)
  data: data function_input double; data function_input double; Pre_x function_input; Pre_vx function_input; Pre_y function_input; Pre_vy function_input; deltaT function_input; pre_p11 function_input; pre_p12 function_input; pre_p13 function_input; pre_p14 function_input; pre_p21 function_input; pre_p22 function_input; pre_p23 function_input; pre_p24 function_input; pre_p31 function_input; pre_p32 function_input; pre_p33 function_input; pre_p34 function_input; pre_p41 function_input; pre_p42 function_input; pre_p43 function_input; pre_p44 function_input; RangeX function_output; VelX function_output; RangeY function_output; VelY function_output; P11 function_output; P12 function_output; P13 function_output; P14 function_output; P21 function_output; P22 function_output; P23 function_output; P24 function_output; P31 function_output; P32 function_output; P33 function_output; P34 function_output; P41 function_output; P42 function_output; P43 function_output; P44 function_output; Pre_x function_input; Pre_vx function_input; Pre_y function_input; Pre_vy function_input; Mea_x function_input; Mea_y function_input; pre_p11 function_input; pre_p12 function_input; pre_p13 function_input; pre_p14 function_input; pre_p21 function_input; pre_p22 function_input; pre_p23 function_input; pre_p24 function_input; pre_p31 function_input; pre_p32 function_input; pre_p33 function_input; pre_p34 function_input; pre_p41 function_input; pre_p42 function_input; pre_p43 function_input; pre_p44 function_input; R11 function_input; R12 function_input; R21 function_input; R22 function_input; RangeX function_output; VelX function_output; RangeY function_output; VelY function_output; P11 function_output; P12 function_output; P13 function_output; P14 function_output; P21 function_output; P22 function_output; P23 function_output; P24 function_output; P31 function_output; P32 function_output; P33 function_output; P34 function_output; P41 function_output; P42 function_output; P43 function_output; P44 function_output; MeasureRx function_input; MeasureRy function_input; PredictRx function_input; PredictRy function_input; P11 function_input; P12 function_input; P13 function_input; P14 function_input; P21 function_input; P22 function_input; P23 function_input; P24 function_input; P31 function_input; P32 function_input; P33 function_input; P34 function_input; P41 function_input; P42 function_input; P43 function_input; P44 function_input; MD function_output; R11 function_input; R12 function_input; R21 function_input; R22 function_input; h temporary double =0; OutSRRFOV function_output double; h temporary double =0; OutESRFOV function_output double; h temporary double =0; OutCameraFOV function_output double; h temporary double =0; Blocked function_output double; x function_input; InPathFlag function_output; y function_input; R function_input double size=1; ESRData input size=[64 4]; FusDataOut output double size=[127 26] =0; MeasureData local double size=[64 11] =0; Num_Trg output double size=1 =0; FusDataInternal_temp local double size=[127 33]; PowerMode local double size=1 =1; DisableCriteria local double size=1 =0; CameraStatus constant double size=1 =1; RadarStatus constant double size=1 =1; DataSource local double size=1; Sensor_sampleTime local double size=1; CameraData input size=[25 8]; n local double size=1 =0; k local double size=1 =0; FusDataInternal local double size=[127 33]; LastCalTime local double size=1 =240; MD_Exist local double size=1 =0; MD_Calib constant double =800; Rx3xgm local double; Ry3xgm local double; MD_min local double size=1 =2000; MeasureFoundFlag local double size=1 =0; MeasureFoundNum local double size=1 =0; UpdateTrackFlag local double size=127 =0; TrackCounter local double size=1 =0; m local double size=1 =0; DelectTrackFlag local double size=127 =0; Num_Out local double size=1 =0; c local double size=1 =0; LastFusID local double size=1 =0; ExistID local double size=1 =0; IDUsedFlag local double size=127 =0; MD_k_m local double size=1 =0; deltaT local double size=1 =0; LoopError local double size=1 =0; SRRData input size=[40 4]; Path_Radius input double; InPathFlag local double; ScoreFlag local double; RollCount output double; CameraFarScoreDe constant double =2; CameraNearScoreDe constant double =5; ESRScoreDe constant double =4; SRRScoreDe constant double =2; SRRScoreIn constant double =4; ESRScoreIn constant double =5; CameraScoreIn constant double =6; ESR_RxTime input double; SRR_RxTime input double; Camera_RxTime input double
  events: cal input EITHER_EDGE_EVENT; cal1 input EITHER_EDGE_EVENT; cal2 input EITHER_EDGE_EVENT

== stateflow chart ADU_Integration_Y2016_simulation/Fusion_Model/Fusion_Block/Side_Fusion/LF_SRR_CoordinateAlig ==
  state [rangeX,rangeY] = TemporalAligLF(range,azimuth,W,L,InstallAngLFSRR) [function]
  (default) -> (junction 95) : {
      | k=0;
      | LFSRR_Output=0;
      | }
  (junction 95) -> (junction 98) [order 1] : [k<10]
  (junction 98) -> (junction 104) [order 1] : [LFSRR_Input[k][0]!=0]
  (junction 101) -> (junction 95) : {
      | k++;
      | }
  (junction 95) -> (junction 96) [order 2] : {
      | SideFusion;
      | }
  (junction 98) -> (junction 101) [order 2]
  (junction 104) -> (junction 106) : {
      | LFSRR_Output[k][0]=LFSRR_Input[k][0];%Target ID
      | [LFSRR_Output[k][1],LFSRR_Output[k][2]]=TemporalAligLF(LFSRR_Input[k][1],LFSRR_Input[k][2],W,L,InstallAng*3.1415/180);
      | LFSRR_Output[k][3]=LFSRR_Input[k][4]; %Target DynamicMode
      | }
  (junction 106) -> (junction 101)
  data: range function_input; rangeX function_output; rangeY function_output; azimuth function_input; W function_input double size=1; L function_input double size=1; InstallAngLFSRR function_input double size=1; LFSRR_Input input double size=[10 5]; LFSRR_Output output double size=[10 4]; k local double size=1 =0; W constant double =1.8; L constant double =5.2; InstallAng constant double =63
  events: SRR_Trig input EITHER_EDGE_EVENT; SideFusion output FUNCTION_CALL_EVENT

== stateflow chart ADU_Integration_Y2016_simulation/Fusion_Model/Fusion_Block/Side_Fusion/LR_SRR_CoordinateAlig ==
  state [rangeX,rangeY] = TemporalAligLR(range,azimuth,W,L,InstallAngLRSRR) [function]
  (default) -> (junction 95) : {
      | k=0;
      | LRSRR_Output=0;
      | }
  (junction 95) -> (junction 98) [order 1] : [k<10]
  (junction 98) -> (junction 104) [order 1] : [LRSRR_Input[k][0]!=0]
  (junction 101) -> (junction 95) : {
      | k++;
      | }
  (junction 95) -> (junction 96) [order 2] : {
      | SideFusion;
      | }
  (junction 98) -> (junction 101) [order 2]
  (junction 104) -> (junction 106) : {
      | LRSRR_Output[k][0]=LRSRR_Input[k][0];%Target ID
      | [LRSRR_Output[k][1],LRSRR_Output[k][2]]=TemporalAligLR(LRSRR_Input[k][1],LRSRR_Input[k][2],W,L,InstallAng*3.1415/180);
      | LRSRR_Output[k][3]=LRSRR_Input[k][4]; %Target DynamicMode
      | }
  (junction 106) -> (junction 101)
  data: range function_input; rangeX function_output; rangeY function_output; azimuth function_input; W function_input double size=1; L function_input double size=1; InstallAngLRSRR function_input double size=1; LRSRR_Input input double size=[10 5]; LRSRR_Output output double size=[10 4]; k local double size=1 =0; L constant double =5.2; W constant double =1.8; InstallAng constant double =60
  events: SRR_Trig input EITHER_EDGE_EVENT; SideFusion output FUNCTION_CALL_EVENT

== stateflow chart ADU_Integration_Y2016_simulation/LogData/Vision_Target/Chart1 ==
  (default) -> (junction 13)
  (junction 13) -> (junction 14) [order 1] : [Trig != preTrig]
  (junction 13) -> (junction 15) [order 2]
  (junction 14) -> (junction 16) : {
      | DataOutput=DataInput;
      | Time_out=Time;
      | }
  (junction 16) -> (junction 15)
  (junction 15) -> (junction 17) : {
      | preTrig=Trig;
      | }
  data: Trig input; Time input; preTrig local double; Time_out output double; DataInput input size=[25 8]; DataOutput output double size=[25 8]

== stateflow chart ADU_Integration_Y2016_simulation/Fusion_Model/Fusion_Block/Side_Fusion/RF_SRR_CoordinateAlig ==
  state [rangeX,rangeY] = TemporalAligRF(range,azimuth,W,L,InstallAngRFSRR) [function]
  (default) -> (junction 95) : {
      | k=0;
      | RFSRR_Output=0;
      | }
  (junction 95) -> (junction 98) [order 1] : [k<10]
  (junction 98) -> (junction 104) [order 1] : [RFSRR_Input[k][0]!=0]
  (junction 101) -> (junction 95) : {
      | k++;
      | }
  (junction 95) -> (junction 96) [order 2] : {
      | SideFusion;
      | }
  (junction 98) -> (junction 101) [order 2]
  (junction 104) -> (junction 106) : {
      | RFSRR_Output[k][0]=RFSRR_Input[k][0];%Target ID
      | [RFSRR_Output[k][1],RFSRR_Output[k][2]]=TemporalAligRF(RFSRR_Input[k][1],RFSRR_Input[k][2],W,L,InstallAng*3.1415/180);
      | RFSRR_Output[k][3]=RFSRR_Input[k][4]; %Target DynamicMode
      | }
  (junction 106) -> (junction 101)
  data: range function_input; rangeX function_output; rangeY function_output; azimuth function_input; W function_input double size=1; L function_input double size=1; InstallAngRFSRR function_input double size=1; RFSRR_Input input double size=[10 5]; RFSRR_Output output double size=[10 4]; k local double size=1 =0; L constant double =5.2; W constant double =1.8; InstallAng constant double =60
  events: SRR_Trig input EITHER_EDGE_EVENT; SideFusion output FUNCTION_CALL_EVENT
